simulink model "DTC_SVM_PI"  (R2020b)
settings: Solver=ode23tb  StartTime=0.0  StopTime=2  FixedStep=1e-5  RelTol=1e-3  EnableMultiTasking=on
libraries: powerlib x4, powerlib_extras x2, simulink x2
settings Model: Creator=Administrator  LastModifiedBy=Ray
settings DataIOCC: LimitDataPoints=on  SaveFormat=Array  SignalLoggingSaveFormat=ModelDataLogs  ReturnWorkspaceOutputs=off
settings OptimizationCC: ExpressionDepthLimit=2147483647  LifeSpan=inf
settings DebuggingCC: UnderspecifiedInitializationDetection=Classic  MergeDetectMultiDrivingBlocksExec=none  SolverPrmCheckMsg=warning  FcnCallInpInsideContextMsg=warning  StateNameClashWarn=warning  SFUnexpectedBacktrackingDiag=warning  SFNoUnconditionalDefaultTransitionDiag=warning  SFExecutionAtInitializationDiag=none  ArithmeticOperatorsInVariantConditions=warning
settings HardwareCC: ProdBitPerPointer=32  ProdBitPerSizeT=32  ProdBitPerPtrDiffT=32  ProdLargestAtomicFloat=None  ProdIntDivRoundTo=Undefined  ProdEndianess=Unspecified  ProdWordSize=32  ProdHWDeviceType=32-bit Generic
settings ModelReferenceCC: PropagateSignalLabelsOutOfModel=off
settings SFSimCC: SimUseLocalCustomCode=off  CustomCodeUndefinedFunction=UseInterfaceOnly
settings RTWCC: RTWUseLocalCustomCode=off
settings CodeAppCC: StateflowObjectComments=on
settings GRTTargetCC: TargetLangStandard=C89/C90 (ANSI)  CombineOutputUpdateFcns=off  GRTInterface=on
settings ConfigComp: CovMetricSettings=dw  CovSaveCumulativeToWorkspaceVar=on  CovSaveSingleToWorkspaceVar=on  CovExternalEMLEnable=off
settings SimscapeCC: SimscapeNormalizeSystem=off

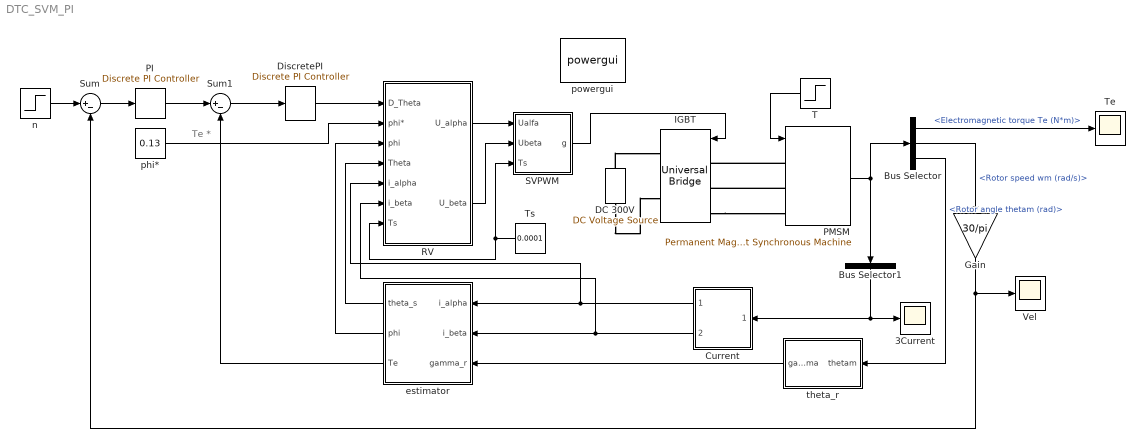
== system DTC_SVM_PI ==
  note: Te *
  3Current : Scope
  Bus Selector : BusSelector  OutputSignals=Electromagnetic torque Te (N*m),Rotor speed wm (rad/s),Rotor angle thetam (rad)
  Bus Selector1 : BusSelector  OutputSignals=Stator current is_a (A),Stator current is_b (A),Stator current is_c (A)  OutputAsBus=on
  "Current " : Subsystem
  DC 300V : powerlib/Electrical Sources/DC Voltage Source  Amplitude=300  Measurements=None
  DiscretePI : powerlib_extras/Discrete  Control Blocks/Discrete PI Controller  Kp=0.08  Ki=0.01  Par_Limits=[0.2 -0.2]  Init=0  Ts=1e-5
  Gain : Gain  Gain=30/pi
  IGBT : powerlib/Power Electronics/Universal Bridge  Arms=3  SnubberResistance=1e5  SnubberCapacitance=inf  Device=IGBT / Diodes  Ron=1e-3  Lon=0  ForwardVoltages="[  0  0  ]"  ForwardVoltage=0  GTOparameters=[ 10e-6 , 20e-6 ]  IGBTparameters=[ 1e-6 , 2e-6 ]  Measurements=None  Measurements_2=None  converterType=Rectifier
  PI : powerlib_extras/Discrete  Control Blocks/Discrete PI Controller  Kp=0.15  Ki=2  Par_Limits=[40 -40]  Init=0  Ts=1e-5
  PMSM : powerlib/Machines/Permanent Magnet Synchronous Machine  NbPhases=3  FluxDistribution=Sinusoidal  RotorType=Salient-pole  MechanicalLoad=Torque Tm  PresetModel=No  ShowDetailedParameters=on  MeasurementBus=off  Resistance=0.0335  Inductance=8.5e-3  dqInductances=[6.4e-3, 6.4e-3]  La=0.000395  MachineConstant=Flux linkage established by magnets (V.s)  Flux=0.13  VoltageCst=94.3176  TorqueCst=0.78  Flat=120  Mechanical=[0.013,0,4]  PolePairs=4  InitialConditions=[0,0, 0,0]  InitialConditions5ph=[0 0 0 0 0 0]  RefAngle=90 degrees behind phase A axis (modified Park)  IterativeDiscreteModel=Trapezoidal non iterative  TsBlock=-1  TsPowergui=0
  RV : Subsystem
  SVPWM : Subsystem
  Sum : Sum  Inputs=|+-
  Sum1 : Sum  Inputs=|+-
  T : Step  After=10  SampleTime=0
  Te : Scope
  Ts : Constant  Value=0.0001
  Vel : Scope
  estimator : Subsystem
  n : Step  Time=0.3  Before=1000  After=1000  SampleTime=0
  phi* : Constant  Value=0.13
  powergui : powerlib/powergui  SimulationMode=Discrete  SampleTime=5e-6  frequency=60  Iterations=50  frequencyindice=0  Pbase=100e6  ErrMax=1e-4  UnitsV=kV  UnitsW=MW  buscounter=0  FunctionMessages=off  echomessages=off  EnableUseOfTLC=off  CurrentSourceSwitches=on  DisableSnubberDevices=off  DisableRonSwitches=off  DisableVfSwitches=off  DisplayEquations=off  AutomaticDiscreteSolvers=off  SolverType=Tustin/Backward Euler (TBE)  Interpol=off  ExternalGateDelay=off  methode=off  Ts=0  x0status=blocks  SPID=off  SwTol=0  HookPort=off  NonlinearTolerance=1e-4  nMaxIteration=100  ContinueOnMaxIteration=off  RestoreLinks=warning  ResistiveCurrentMeasurement=off  Frange=[0:2:500]  Ylog=off  Xlog=on  ShowGrid=off  save=off  variable=ZData  structure=0  ZoomFFT=on  StartTime=0.0  cycles=1  DisplayStyle=1  fundamental=60  FreqAxis=off  MaxFrequency=1000  frequencyindicesteady=1  RmsSteady=1  display=off
  theta_r : Subsystem
  wires:
  PMSM/1 -> Bus Selector/1, Bus Selector1/1
  T/1 -> PMSM/1
  n/1 -> Sum/1
  PI/1 -> Sum1/1
  Sum1/1 -> DiscretePI/1
  Bus Selector/2 -> Gain/1  "<Rotor speed wm (rad/s)>"
  estimator/3(Te) -> Sum1/2
  DiscretePI/1 -> RV/1(D_Theta)
  phi*/1 -> RV/2(phi*)
  estimator/2(phi) -> RV/3(phi)
  estimator/1(theta_s) -> RV/4(Theta)
  Bus Selector/1 -> Te/1  "<Electromagnetic torque Te (N*m)>"
  Gain/1 -> Vel/1, Sum/2
  "Current "/1(i_alpa) -> estimator/1(i_alpha), RV/5(i_alpha)
  "Current "/2(i_beta) -> estimator/2(i_beta), RV/6(i_beta)
  RV/2(U_beta) -> SVPWM/2(Ubeta)
  RV/1(U_alpha) -> SVPWM/1(Ualfa)
  SVPWM/1(g) -> IGBT/1
  Bus Selector/3 -> theta_r/1(thetam)  "<Rotor angle thetam (rad)>"
  theta_r/1(gamma) -> estimator/3(gamma_r)
  Sum/1 -> PI/1
  Ts/1 -> SVPWM/3(Ts), RV/7(Ts)
  Bus Selector1/1 -> 3Current/1, "Current "/1(i_abc)
  connections:
  PMSM/LConn2 -- IGBT/LConn2
  IGBT/LConn3 -- PMSM/LConn3
  DC 300V/RConn1 -- IGBT/RConn1
  DC 300V/LConn1 -- IGBT/RConn2
  PMSM/LConn1 -- IGBT/LConn1

== system DTC_SVM_PI/Current  ==
  i_abc : Inport
  Fcn : Fcn  Expr=(2/3)^0.5*(u(1)-u(2)/2-u(3)/2)
  Fcn1 : Fcn  Expr=(2/3)^0.5*(sqrt(3)/2)*(u(2)-u(3))
  i_alpa : Outport
  i_beta : Outport  Port=2
  wires:
  Fcn/1 -> i_alpa/1
  Fcn1/1 -> i_beta/1
  i_abc/1 -> Fcn/1, Fcn1/1

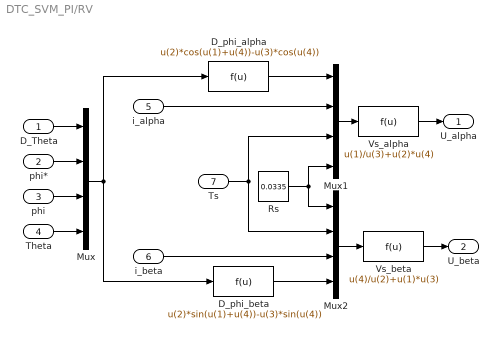
== system DTC_SVM_PI/RV ==
  D_Theta : Inport
  phi* : Inport  Port=2
  phi : Inport  Port=3
  Theta : Inport  Port=4
  i_alpha : Inport  Port=5
  i_beta : Inport  Port=6
  Ts : Inport  Port=7
  " Rs" : Constant  Value=0.0335
  D_phi_alpha : Fcn  Expr=u(2)*cos(u(1)+u(4))-u(3)*cos(u(4))
  D_phi_beta : Fcn  Expr=u(2)*sin(u(1)+u(4))-u(3)*sin(u(4))
  Mux : Mux
  Mux1 : Mux
  Mux2 : Mux
  Vs_alpha : Fcn  Expr=u(1)/u(3)+u(2)*u(4)
  Vs_beta : Fcn  Expr=u(4)/u(2)+u(1)*u(3)
  U_alpha : Outport
  U_beta : Outport  Port=2
  wires:
  Vs_alpha/1 -> U_alpha/1
  Vs_beta/1 -> U_beta/1
  D_Theta/1 -> Mux/1
  phi*/1 -> Mux/2
  phi/1 -> Mux/3
  Theta/1 -> Mux/4
  Mux/1 -> D_phi_alpha/1, D_phi_beta/1
  D_phi_alpha/1 -> Mux1/1
  i_alpha/1 -> Mux1/2
  D_phi_beta/1 -> Mux2/4
  i_beta/1 -> Mux2/3
  Ts/1 -> Mux1/3, Mux2/2
  " Rs"/1 -> Mux1/4, Mux2/1
  Mux1/1 -> Vs_alpha/1
  Mux2/1 -> Vs_beta/1

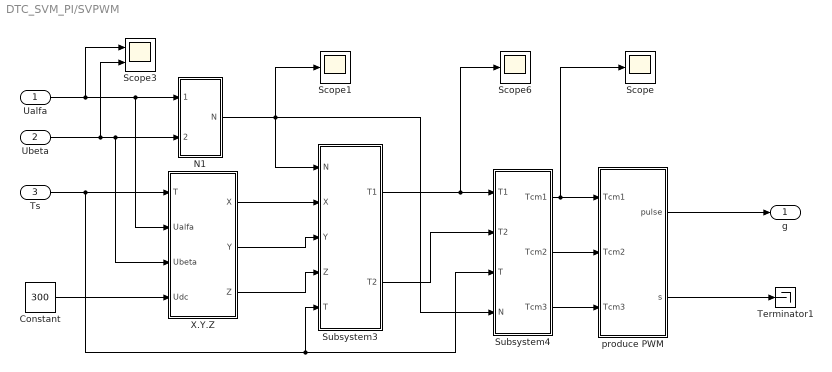
== system DTC_SVM_PI/SVPWM ==
  Ualfa : Inport
  Ubeta : Inport  Port=2
  Ts : Inport  Port=3
  Constant : Constant  Value=300
  N1 : Subsystem
  Scope : Scope
  Scope1 : Scope
  Scope3 : Scope  NumInputPorts=2
  Scope6 : Scope
  Subsystem3 : Subsystem
  Subsystem4 : Subsystem
  Terminator1 : Terminator
  X.Y.Z : Subsystem
  produce PWM : Subsystem
  g : Outport
  wires:
  Ts/1 -> X.Y.Z/1(T), Subsystem4/3(T), Subsystem3/5(T)
  Constant/1 -> X.Y.Z/4(Udc)
  N1/1(N) -> Subsystem4/4(N), Scope1/1, Subsystem3/1(N)
  X.Y.Z/1(X) -> Subsystem3/2(X)
  X.Y.Z/2(Y) -> Subsystem3/3(Y)
  X.Y.Z/3(Z) -> Subsystem3/4(Z)
  Subsystem4/1(Tcm1) -> produce PWM/1(Tcm1), Scope/1
  Subsystem4/2(Tcm2) -> produce PWM/2(Tcm2)
  Subsystem4/3(Tcm3) -> produce PWM/3(Tcm3)
  Ualfa/1 -> Scope3/1, X.Y.Z/2(Ualfa), N1/1(Ualfa)
  Subsystem3/1(T1) -> Subsystem4/1(T1), Scope6/1
  Subsystem3/2(T2) -> Subsystem4/2(T2)
  Ubeta/1 -> N1/2(Ubeta), X.Y.Z/3(Ubeta), Scope3/2
  produce PWM/1(pulse) -> g/1
  produce PWM/2(s) -> Terminator1/1

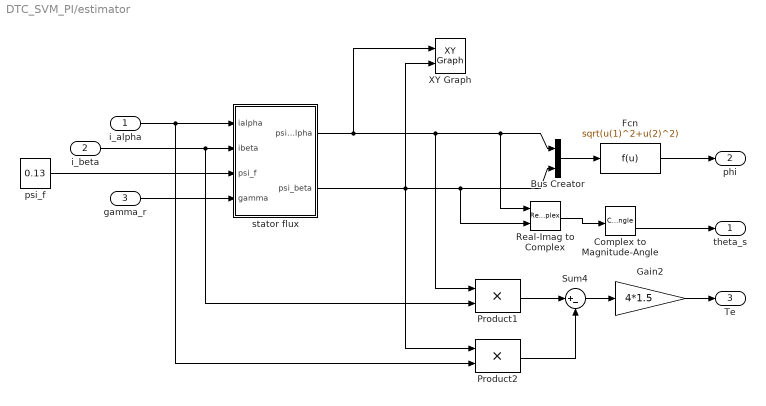
== system DTC_SVM_PI/estimator ==
  i_alpha : Inport
  i_beta : Inport  Port=2
  gamma_r : Inport  Port=3
  Bus Creator : BusCreator  Inputs=2
  Complex to Magnitude-Angle : ComplexToMagnitudeAngle
  Fcn : Fcn  Expr=sqrt(u(1)^2+u(2)^2)
  Gain2 : Gain  Gain=4*1.5  SaturateOnIntegerOverflow=on  OutDataTypeStr=Inherit: Same as input  ParamDataTypeStr=Inherit: Same as input
  Product1 : Product  SaturateOnIntegerOverflow=on  OutDataTypeStr=Inherit: Same as first input
  Product2 : Product  SaturateOnIntegerOverflow=on  OutDataTypeStr=Inherit: Same as first input
  Real-Imag to Complex : RealImagToComplex
  Sum4 : Sum  Inputs=|+-  SaturateOnIntegerOverflow=on
  XY Graph : simulink/Sinks/XY Graph  xmin=-0.2  xmax=0.2  ymin=-0.2  ymax=0.2  st=-1
  psi_f : Constant  Value=0.13
  stator flux : Subsystem
  theta_s : Outport
  phi : Outport  Port=2
  Te : Outport  Port=3
  wires:
  Product1/1 -> Sum4/1
  Product2/1 -> Sum4/2
  Sum4/1 -> Gain2/1
  Complex to Magnitude-Angle/2 -> theta_s/1
  Gain2/1 -> Te/1
  gamma_r/1 -> stator flux/4(gamma)
  psi_f/1 -> stator flux/3(psi_f)
  stator flux/1(psi_alpha) -> XY Graph/1, Product1/1, Real-Imag to Complex/1, Bus Creator/1
  stator flux/2(psi_beta) -> Product2/1, XY Graph/2, Real-Imag to Complex/2, Bus Creator/2
  i_alpha/1 -> stator flux/1(ialpha), Product2/2
  i_beta/1 -> stator flux/2(ibeta), Product1/2
  Bus Creator/1 -> Fcn/1
  Fcn/1 -> phi/1
  Real-Imag to Complex/1 -> Complex to Magnitude-Angle/1

== system DTC_SVM_PI/theta_r ==
  thetam : Inport
  Add2 : Sum
  const : Constant  Value=3*pi/2
  np=4 : Gain  Gain=4
  gamma : Outport
  wires:
  thetam/1 -> np=4/1
  Add2/1 -> gamma/1
  const/1 -> Add2/1
  np=4/1 -> Add2/2

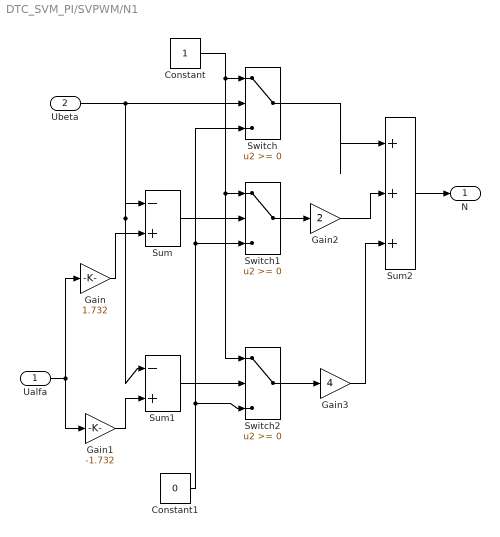
== system DTC_SVM_PI/SVPWM/N1 ==
  Ualfa : Inport
  Ubeta : Inport  Port=2
  Constant : Constant
  Constant1 : Constant  Value=0
  Gain : Gain  Gain=1.732
  Gain1 : Gain  Gain=-1.732
  Gain2 : Gain  Gain=2
  Gain3 : Gain  Gain=4
  Sum : Sum  Inputs=|-+
  Sum1 : Sum  Inputs=|-+
  Sum2 : Sum  Inputs=|+++
  Switch : Switch
  Switch1 : Switch
  Switch2 : Switch
  N : Outport
  wires:
  Ubeta/1 -> Switch/2, Sum/1, Sum1/1
  Constant/1 -> Switch/1, Switch2/1, Switch1/1
  Ualfa/1 -> Gain1/1, Gain/1
  Gain/1 -> Sum/2
  Sum/1 -> Switch1/2
  Sum1/1 -> Switch2/2
  Gain1/1 -> Sum1/2
  Constant1/1 -> Switch/3, Switch1/3, Switch2/3
  Switch1/1 -> Gain2/1
  Switch2/1 -> Gain3/1
  Gain2/1 -> Sum2/2
  Switch/1 -> Sum2/1
  Gain3/1 -> Sum2/3
  Sum2/1 -> N/1

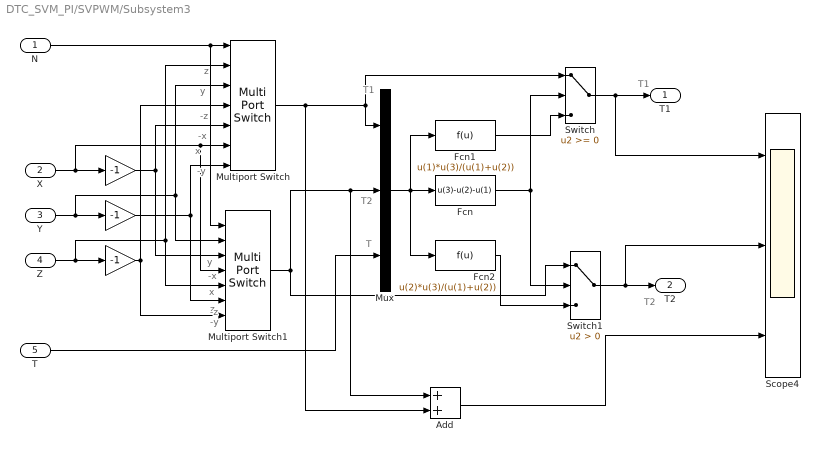
== system DTC_SVM_PI/SVPWM/Subsystem3 ==
  note: z
  note: y
  note: -z
  note: -x
  note: x
  note: -y
  note: y
  note: -x
  note: x
  note: z
  note: -y
  note: -z
  note: T1
  note: T2
  note: T
  note: T1
  note: T2
  N : Inport
  X : Inport  Port=2
  Y : Inport  Port=3
  Z : Inport  Port=4
  T : Inport  Port=5
  " " : Gain  Gain=-1
  "  " : Gain  Gain=-1
  "    " : Gain  Gain=-1
  Add : Sum
  Fcn : Fcn  Expr=u(3)-u(2)-u(1)
  Fcn1 : Fcn  Expr=u(1)*u(3)/(u(1)+u(2))
  Fcn2 : Fcn  Expr=u(2)*u(3)/(u(1)+u(2))
  Multiport Switch : MultiPortSwitch  Inputs=6
  Multiport Switch1 : MultiPortSwitch  Inputs=6
  Mux : Mux  Inputs=3
  Scope4 : Scope  NumInputPorts=3
  Switch : Switch
  Switch1 : Switch  Criteria=u2 > Threshold
  T1 : Outport
  T2 : Outport  Port=2
  wires:
  N/1 -> Multiport Switch1/1, Multiport Switch/1
  X/1 -> Multiport Switch1/4, Multiport Switch/6, " "/1
  Y/1 -> Multiport Switch1/2, Multiport Switch/3, "  "/1
  Z/1 -> Multiport Switch1/5, Multiport Switch/2, "    "/1
  "    "/1 -> Multiport Switch1/7, Multiport Switch/4
  "  "/1 -> Multiport Switch/7, Multiport Switch1/6
  " "/1 -> Multiport Switch/5, Multiport Switch1/3
  Multiport Switch/1 -> Mux/1, Switch/1, Add/2
  Multiport Switch1/1 -> Switch1/1, Mux/2, Add/1
  T/1 -> Mux/3
  Mux/1 -> Fcn/1, Fcn1/1, Fcn2/1
  Fcn/1 -> Switch/2, Switch1/2
  Fcn1/1 -> Switch/3
  Fcn2/1 -> Switch1/3
  Switch/1 -> T1/1, Scope4/1
  Switch1/1 -> T2/1, Scope4/2
  Add/1 -> Scope4/3

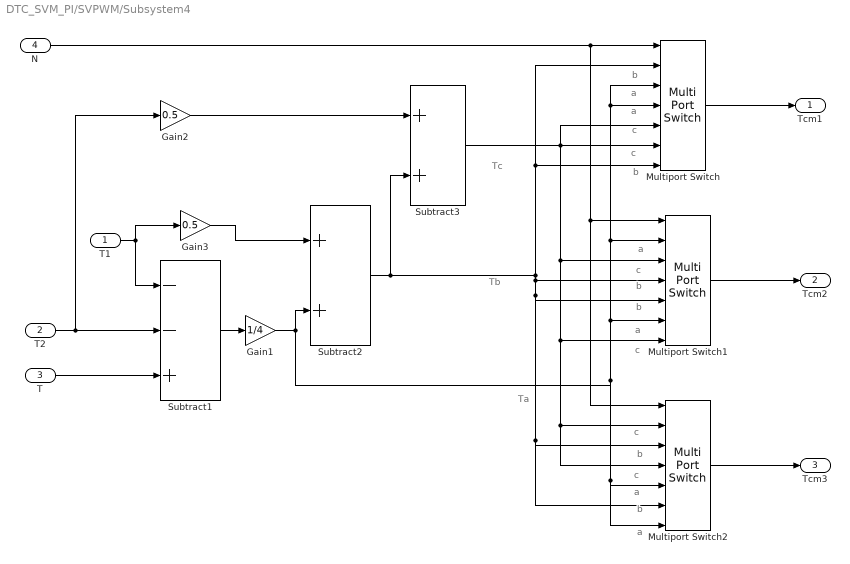
== system DTC_SVM_PI/SVPWM/Subsystem4 ==
  note: Ta
  note: Tb
  note: Tc
  note: b
  note: a
  note: a
  note: c
  note: c
  note: b
  note: a
  note: c
  note: b
  note: b
  note: a
  note: c
  note: c
  note: b
  note: c
  note: a
  note: b
  note: a
  T1 : Inport
  T2 : Inport  Port=2
  T : Inport  Port=3
  N : Inport  Port=4
  Gain1 : Gain  Gain=1/4
  Gain2 : Gain  Gain=0.5
  Gain3 : Gain  Gain=0.5
  Multiport Switch : MultiPortSwitch  Inputs=6
  Multiport Switch1 : MultiPortSwitch  Inputs=6
  Multiport Switch2 : MultiPortSwitch  Inputs=6
  Subtract1 : Sum  Inputs=--+
  Subtract2 : Sum
  Subtract3 : Sum
  Tcm1 : Outport
  Tcm2 : Outport  Port=2
  Tcm3 : Outport  Port=3
  wires:
  T2/1 -> Gain2/1, Subtract1/2
  T/1 -> Subtract1/3
  T1/1 -> Gain3/1, Subtract1/1
  Gain3/1 -> Subtract2/1
  Subtract1/1 -> Gain1/1
  Gain1/1 -> Subtract2/2, Multiport Switch/3, Multiport Switch/4, Multiport Switch1/2, Multiport Switch1/6, Multiport Switch2/5, Multiport Switch2/7
  Subtract2/1 -> Subtract3/2, Multiport Switch/2, Multiport Switch/7, Multiport Switch1/4, Multiport Switch1/5, Multiport Switch2/3, Multiport Switch2/6
  Gain2/1 -> Subtract3/1
  N/1 -> Multiport Switch/1, Multiport Switch2/1, Multiport Switch1/1
  Multiport Switch/1 -> Tcm1/1
  Multiport Switch1/1 -> Tcm2/1
  Multiport Switch2/1 -> Tcm3/1
  Subtract3/1 -> Multiport Switch/5, Multiport Switch/6, Multiport Switch1/3, Multiport Switch1/7, Multiport Switch2/2, Multiport Switch2/4

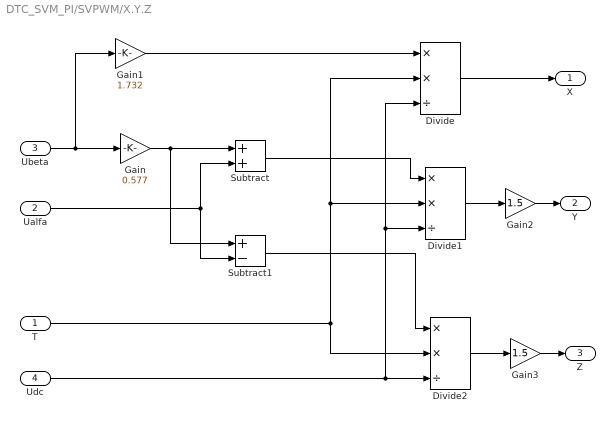
== system DTC_SVM_PI/SVPWM/X.Y.Z ==
  T : Inport
  Ualfa : Inport  Port=2
  Ubeta : Inport  Port=3
  Udc : Inport  Port=4
  Divide : Product  Inputs=**/
  Divide1 : Product  Inputs=**/
  Divide2 : Product  Inputs=**/
  Gain : Gain  Gain=0.577
  Gain1 : Gain  Gain=1.732
  Gain2 : Gain  Gain=1.5
  Gain3 : Gain  Gain=1.5
  Subtract : Sum
  Subtract1 : Sum  Inputs=+-
  X : Outport
  Y : Outport  Port=2
  Z : Outport  Port=3
  wires:
  Gain/1 -> Subtract/1, Subtract1/1
  Gain1/1 -> Divide/1
  T/1 -> Divide2/2, Divide1/2, Divide/2
  Udc/1 -> Divide2/3, Divide1/3, Divide/3
  Ualfa/1 -> Subtract1/2, Subtract/2
  Subtract/1 -> Divide1/1
  Subtract1/1 -> Divide2/1
  Divide/1 -> X/1
  Divide1/1 -> Gain2/1
  Divide2/1 -> Gain3/1
  Gain2/1 -> Y/1
  Gain3/1 -> Z/1
  Ubeta/1 -> Gain1/1, Gain/1

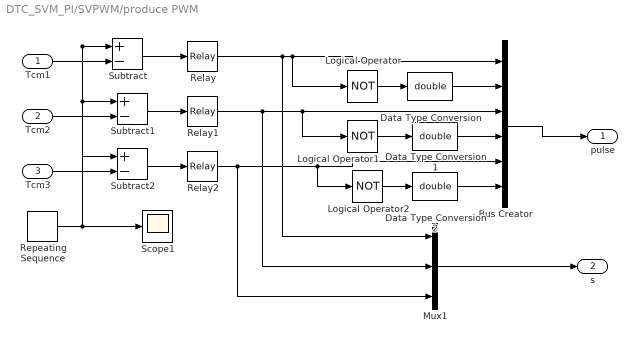
== system DTC_SVM_PI/SVPWM/produce PWM ==
  Tcm1 : Inport
  Tcm2 : Inport  Port=2
  Tcm3 : Inport  Port=3
  Bus Creator : BusCreator  Inputs=6
  Data Type Conversion : DataTypeConversion  OutDataTypeStr=double
  Data Type Conversion1 : DataTypeConversion  OutDataTypeStr=double
  Data Type Conversion2 : DataTypeConversion  OutDataTypeStr=double
  Logical Operator : Logic  Operator=NOT  AllPortsSameDT=off
  Logical Operator1 : Logic  Operator=NOT  AllPortsSameDT=off
  Logical Operator2 : Logic  Operator=NOT  AllPortsSameDT=off
  Mux1 : Mux  Inputs=3
  Relay : Relay
  Relay1 : Relay
  Relay2 : Relay
  Repeating Sequence : simulink/Sources/Repeating Sequence  rep_seq_t=[0 0.00005 0.0001]  rep_seq_y=[0 0.00005 0]
  Scope1 : Scope
  Subtract : Sum  Inputs=+-
  Subtract1 : Sum  Inputs=+-
  Subtract2 : Sum  Inputs=+-
  pulse : Outport
  s : Outport  Port=2
  wires:
  Subtract/1 -> Relay/1
  Subtract1/1 -> Relay1/1
  Subtract2/1 -> Relay2/1
  Repeating Sequence/1 -> Subtract/1, Subtract2/1, Subtract1/1, Scope1/1
  Tcm1/1 -> Subtract/2
  Tcm2/1 -> Subtract1/2
  Tcm3/1 -> Subtract2/2
  Logical Operator1/1 -> Data Type Conversion1/1
  Logical Operator2/1 -> Data Type Conversion2/1
  Logical Operator/1 -> Data Type Conversion/1
  Relay/1 -> Bus Creator/1, Logical Operator/1, Mux1/1
  Relay1/1 -> Bus Creator/3, Logical Operator1/1, Mux1/2
  Relay2/1 -> Bus Creator/5, Logical Operator2/1, Mux1/3
  Bus Creator/1 -> pulse/1
  Data Type Conversion/1 -> Bus Creator/2
  Data Type Conversion1/1 -> Bus Creator/4
  Data Type Conversion2/1 -> Bus Creator/6
  Mux1/1 -> s/1

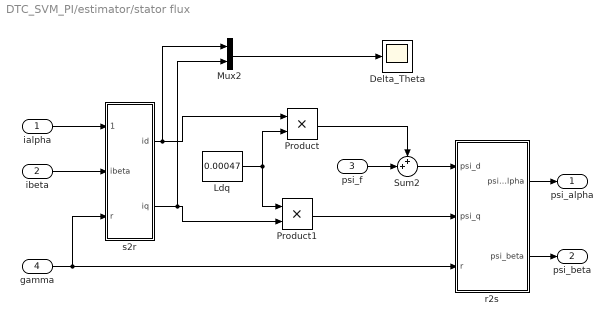
== system DTC_SVM_PI/estimator/stator flux ==
  ialpha : Inport
  ibeta : Inport  Port=2
  psi_f : Inport  Port=3
  gamma : Inport  Port=4
  Delta_Theta : Scope
  Ldq : Constant  Value=0.00047
  Mux2 : Mux  Inputs=2
  Product : Product  RndMeth=Zero
  Product1 : Product  RndMeth=Zero
  Sum2 : Sum  Inputs=++|
  r2s : Subsystem
  s2r : Subsystem
  psi_alpha : Outport
  psi_beta : Outport  Port=2
  wires:
  s2r/1(id) -> Product/1, Mux2/1
  Ldq/1 -> Product/2, Product1/1
  ialpha/1 -> s2r/1(ialpha)
  ibeta/1 -> s2r/2(ibeta)
  gamma/1 -> s2r/3(r), r2s/3(r)
  Product1/1 -> r2s/2(psi_q)
  psi_f/1 -> Sum2/2
  Product/1 -> Sum2/1
  Sum2/1 -> r2s/1(psi_d)
  r2s/1(psi_alpha) -> psi_alpha/1
  r2s/2(psi_beta) -> psi_beta/1
  s2r/2(iq) -> Product1/2, Mux2/2
  Mux2/1 -> Delta_Theta/1

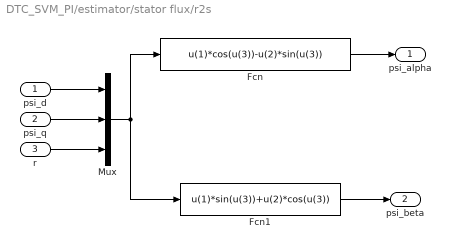
== system DTC_SVM_PI/estimator/stator flux/r2s ==
  psi_d : Inport
  psi_q : Inport  Port=2
  r : Inport  Port=3
  Fcn : Fcn  Expr=u(1)*cos(u(3))-u(2)*sin(u(3))
  Fcn1 : Fcn  Expr=u(1)*sin(u(3))+u(2)*cos(u(3))
  Mux : Mux  Inputs=3
  psi_alpha : Outport
  psi_beta : Outport  Port=2
  wires:
  Fcn/1 -> psi_alpha/1
  psi_d/1 -> Mux/1
  psi_q/1 -> Mux/2
  r/1 -> Mux/3
  Mux/1 -> Fcn1/1, Fcn/1
  Fcn1/1 -> psi_beta/1

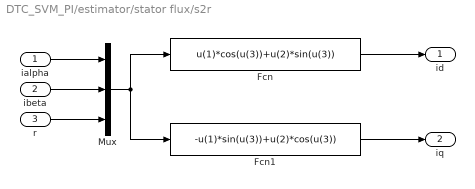
== system DTC_SVM_PI/estimator/stator flux/s2r ==
  ialpha : Inport
  ibeta : Inport  Port=2
  r : Inport  Port=3
  Fcn : Fcn  Expr=u(1)*cos(u(3))+u(2)*sin(u(3))
  Fcn1 : Fcn  Expr=-u(1)*sin(u(3))+u(2)*cos(u(3))
  Mux : Mux  Inputs=3
  id : Outport
  iq : Outport  Port=2
  wires:
  Fcn1/1 -> iq/1
  Fcn/1 -> id/1
  ialpha/1 -> Mux/1
  ibeta/1 -> Mux/2
  r/1 -> Mux/3
  Mux/1 -> Fcn/1, Fcn1/1
